simulink subsystem "coeff_bank_single_ram"  (R2021b)
settings: Solver=VariableStepAuto  StartTime=0.0  StopTime=10.0  RelTol=1e-3
libraries: simulink x1, hdlsllib x1
settings Model: Creator=torha  LastModifiedBy=torha
settings SolverCC: AlgebraicLoopSolver=TrustRegion
settings DebuggingCC: SFMachineParentedDataDiag=warning

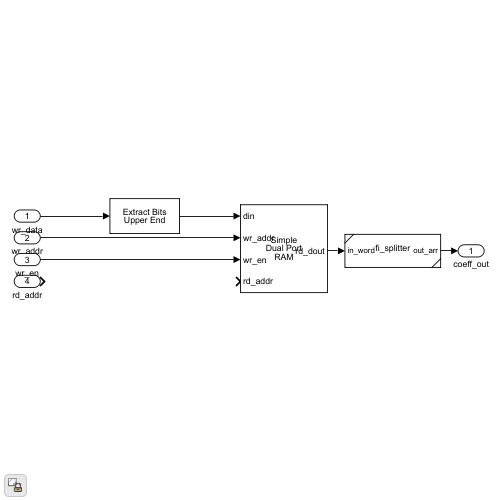
[thumbnail: Simulink's stored preview of the top-level diagram]
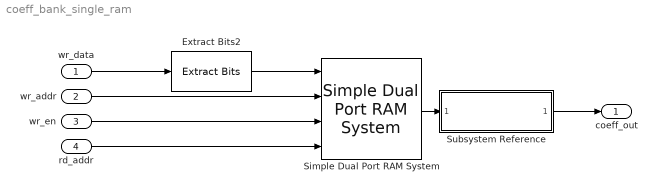
== system coeff_bank_single_ram ==
  wr_data : Inport
  wr_addr : Inport  Port=2
  wr_en : Inport  Port=3
  rd_addr : Inport  Port=4
  Extract Bits2 : simulink/Logic and Bit Operations/Extract Bits  bitsToExtract=Range starting with most significant bit  numBits=last_ram_size  bitIdxRange=[0 7]  outScalingMode=Treat bit field as an integer
  Simple Dual Port RAM System : hdlsllib/HDL RAMs/Simple Dual Port RAM System  RAMType=Simple dual port  WriteOutputValue=New data  RAMInitialValue=0  SimulateUsing=Code generation
      settings: SourceProductBaseCode=SL
  Subsystem Reference : Subsystem  ReferencedSubsystem=fi_splitter  in_bitwidth=last_ram_size  out_bitwidth=coeff.coeff_bitwidth
  coeff_out : Outport
  wires:
  Subsystem Reference/1 -> coeff_out/1
  wr_addr/1 -> Simple Dual Port RAM System/2
  Simple Dual Port RAM System/1 -> Subsystem Reference/1
  Extract Bits2/1 -> Simple Dual Port RAM System/1
  wr_en/1 -> Simple Dual Port RAM System/3
  wr_data/1 -> Extract Bits2/1
  rd_addr/1 -> Simple Dual Port RAM System/4
